simulink library "bouyancyCalculator_ul"  (R2018b)
settings: Solver=VariableStepAuto  StartTime=0.0  StopTime=10.0  RelTol=1e-3
values from neighbouring files (symbols this model uses):
  D = sum(normalVecMat'.*relVelGnd',2)    [oceanForceFunct.m]
  gndStn = OCT.sixDoFStation    [groundStation001_ts3.m]
libraries: vrlib x1
settings Model: Creator=jcreed2  LastModifiedBy=jcreed2

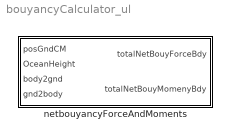
== system bouyancyCalculator_ul ==
  netbouyancyForceAndMoments : Subsystem

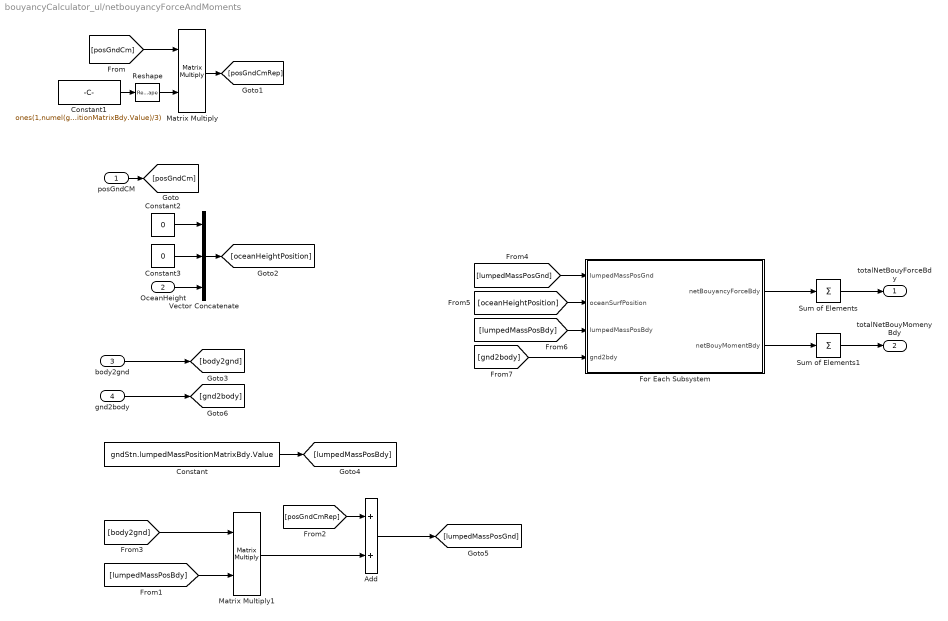
== system bouyancyCalculator_ul/netbouyancyForceAndMoments ==
  posGndCM : Inport
  OceanHeight : Inport  Port=2
  body2gnd : Inport  Port=3
  "gnd2body " : Inport  Port=4
  Add : Sum
  Constant : Constant  Value=gndStn.lumpedMassPositionMatrixBdy.Value
  Constant1 : Constant  Value=ones(1,numel(gndStn.lumpedMassPositionMatrixBdy.Value)/3)
  Constant2 : Constant  Value=0
  Constant3 : Constant  Value=0
  For Each Subsystem : Subsystem  TreatAsAtomicUnit=on  mask{mR=5, netBouy=gndStn.lumpedMassNetBouyancyForce.Value'}
      mask prompts: mR "lumped mass radius"; netBouy "net bouyancy per lumped mass"
  Matrix Multiply : Product  Multiplication=Matrix(*)
  Matrix Multiply1 : Product  Multiplication=Matrix(*)
  Reshape : Reshape  OutputDimensionality=Row vector (2-D)
  Sum of Elements : Sum  Inputs=+
  Sum of Elements1 : Sum  Inputs=+
  Vector Concatenate : Concatenate  NumInputs=3
  totalNetBouyForceBdy : Outport
  totalNetBouyMomenyBdy : Outport  Port=2
  wires:
  Constant2/1 -> Vector Concatenate/1
  [lumpedMassPosBdy] -> Matrix Multiply1/2
  Matrix Multiply/1 -> [posGndCmRep]
  For Each Subsystem/2(netBouyMomentBdy) -> Sum of Elements1/1
  [gnd2body] -> For Each Subsystem/4("gnd2bdy ")
  Vector Concatenate/1 -> [oceanHeightPosition]
  [oceanHeightPosition] -> For Each Subsystem/2(oceanSurfPosition)
  [lumpedMassPosGnd] -> For Each Subsystem/1(lumpedMassPosGnd)
  body2gnd/1 -> [body2gnd]
  OceanHeight/1 -> Vector Concatenate/3
  [body2gnd] -> Matrix Multiply1/1
  Add/1 -> [lumpedMassPosGnd]
  Constant1/1 -> Reshape/1
  [posGndCmRep] -> Add/1
  Sum of Elements1/1 -> totalNetBouyMomenyBdy/1
  Constant3/1 -> Vector Concatenate/2
  [posGndCm] -> Matrix Multiply/1
  Constant/1 -> [lumpedMassPosBdy]
  Matrix Multiply1/1 -> Add/2
  "gnd2body "/1 -> [gnd2body]
  Sum of Elements/1 -> totalNetBouyForceBdy/1
  posGndCM/1 -> [posGndCm]
  For Each Subsystem/1(netBouyancyForceBdy) -> Sum of Elements/1
  [lumpedMassPosBdy] -> For Each Subsystem/3(lumpedMassPosBdy)
  Reshape/1 -> Matrix Multiply/2

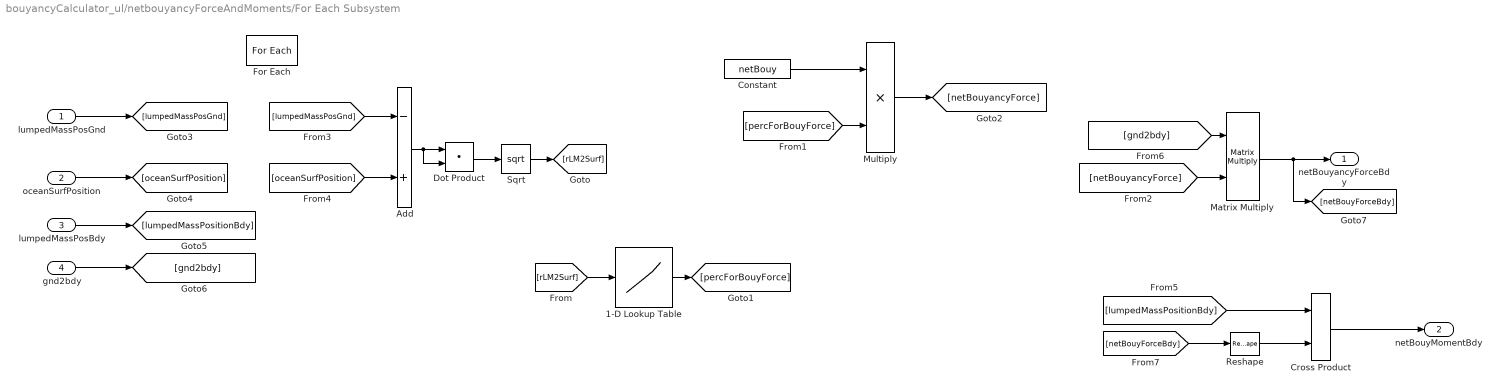
== system bouyancyCalculator_ul/netbouyancyForceAndMoments/For Each Subsystem ==
  lumpedMassPosGnd : Inport  Partition=on  PartitionDimension=2  PartitionWidth=1  PartitionOffset=0
  oceanSurfPosition : Inport  Port=2
  lumpedMassPosBdy : Inport  Port=3  Partition=on  PartitionDimension=2  PartitionWidth=1  PartitionOffset=0
  "gnd2bdy " : Inport  Port=4
  1-D Lookup Table : Lookup_n-D  NumberOfTableDimensions=1  BreakpointsForDimension1=[-mR, .5*-mR, 0, .5*mR, mR]  Table=[0, .25, .5 ,.75,1]  ExtrapMethod=Clip  InternalRulePriority=Speed  RndMeth=Simplest  InputSameDT=on
  Add : Sum  Inputs=-+
  Constant : Constant  Value=netBouy
  Cross Product : vrlib/Utilities/Cross Product
      settings: SourceProductBaseCode=VR
  Dot Product : DotProduct  InputSameDT=on  OutDataTypeStr=Inherit: Inherit via internal rule
  For Each : ForEach  DisableCoverage=on  IndexMode=One-based
  Matrix Multiply : Product  Multiplication=Matrix(*)
  Multiply : Product
  Reshape : Reshape  OutputDimensionality=Column vector (2-D)
  Sqrt : Sqrt  SaturateOnIntegerOverflow=on
  netBouyancyForceBdy : Outport  ConcatenationDimension=1
  netBouyMomentBdy : Outport  Port=2  ConcatenationDimension=1
  wires:
  oceanSurfPosition/1 -> [oceanSurfPosition]
  lumpedMassPosGnd/1 -> [lumpedMassPosGnd]
  Add/1 -> Dot Product/2, Dot Product/1
  Dot Product/1 -> Sqrt/1
  Sqrt/1 -> [rLM2Surf]
  [rLM2Surf] -> 1-D Lookup Table/1
  1-D Lookup Table/1 -> [percForBouyForce]
  [percForBouyForce] -> Multiply/2
  Constant/1 -> Multiply/1
  Multiply/1 -> [netBouyancyForce]
  [netBouyancyForce] -> Matrix Multiply/2
  [lumpedMassPosGnd] -> Add/1
  [oceanSurfPosition] -> Add/2
  [lumpedMassPositionBdy] -> Cross Product/1
  lumpedMassPosBdy/1 -> [lumpedMassPositionBdy]
  "gnd2bdy "/1 -> [gnd2bdy]
  [gnd2bdy] -> Matrix Multiply/1
  Matrix Multiply/1 -> [netBouyForceBdy], netBouyancyForceBdy/1
  [netBouyForceBdy] -> Reshape/1
  Cross Product/1 -> netBouyMomentBdy/1
  Reshape/1 -> Cross Product/2
